simulink model "simple_cosimulation"  (R2021b)
settings: Solver=ode45  StartTime=0.0  StopTime=15  FixedStep=0.01  RelTol=1e-3  EnableMultiTasking=on
libraries: instrumentlib x2, simulink x1
settings Model: PacingRate=11  Creator=tasora  LastModifiedBy=Trevor
settings SolverCC: AlgebraicLoopSolver=TrustRegion
settings DataIOCC: LimitDataPoints=on  SaveFormat=Array  SignalLoggingSaveFormat=ModelDataLogs  ReturnWorkspaceOutputs=off
settings OptimizationCC: ExpressionDepthLimit=2147483647  LifeSpan=inf
settings DebuggingCC: UnderspecifiedInitializationDetection=Classic  MergeDetectMultiDrivingBlocksExec=none  SolverPrmCheckMsg=warning  FcnCallInpInsideContextMsg=warning  StateNameClashWarn=warning  SFUnexpectedBacktrackingDiag=warning  SFNoUnconditionalDefaultTransitionDiag=warning  SFExecutionAtInitializationDiag=none  SFMachineParentedDataDiag=warning  ArithmeticOperatorsInVariantConditions=warning
settings HardwareCC: ProdBitPerPointer=32  ProdBitPerSizeT=32  ProdBitPerPtrDiffT=32  ProdLargestAtomicFloat=None  ProdIntDivRoundTo=Undefined  ProdEndianess=Unspecified  ProdWordSize=32  ProdHWDeviceType=32-bit Generic
settings ModelReferenceCC: PropagateSignalLabelsOutOfModel=off
settings SFSimCC: SimUseLocalCustomCode=off  CustomCodeUndefinedFunction=UseInterfaceOnly
settings RTWCC: RTWUseLocalCustomCode=off
settings CodeAppCC: StateflowObjectComments=on
settings GRTTargetCC: TargetLangStandard=C89/C90 (ANSI)  CombineOutputUpdateFcns=off  GRTInterface=on
settings ConfigComp: CovMetricSettings=dw  CovSaveCumulativeToWorkspaceVar=on  CovSaveSingleToWorkspaceVar=on  CovExternalEMLEnable=off

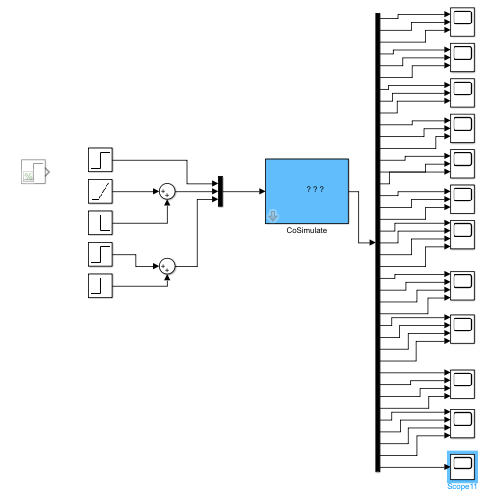
[thumbnail: Simulink's stored preview of the top-level diagram]
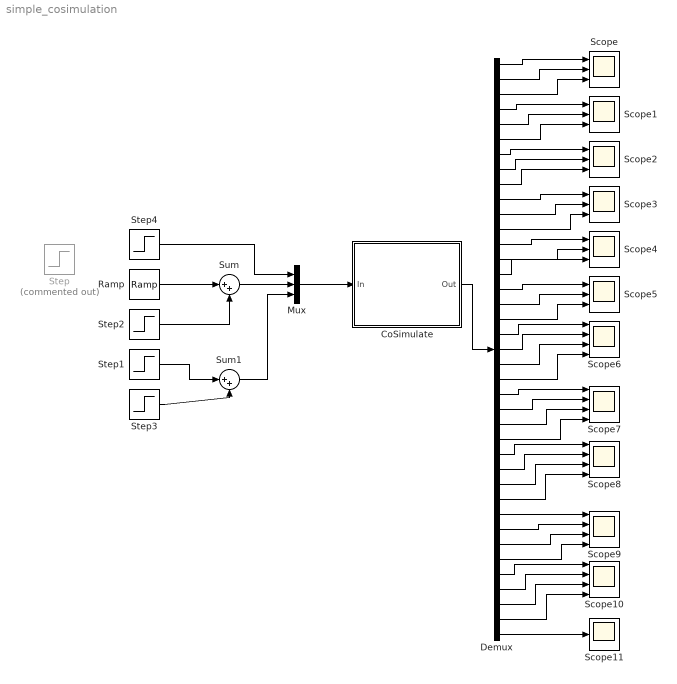
== system simple_cosimulation ==
  CoSimulate : Subsystem  Description=|  mask{com_step=1e-2, tcp_data_size=39, host_name=localhost, tcp_port=50009, tcp_timeout=5}
      | This block can be used to exchange data with Chrono::Engine.                                                                                      
      | A Chrono::Engine program with a running ChCosimulation inferface must be started, it will work as a server; then the Simulink program must be run.
      | Note! check that the dimensions of the exchanged vectors do match!
      mask prompts: com_step "Communication step size"; tcp_data_size "N. of scalars received from C::E (as block output)"; host_name "TCP host name (ex. 'localhost', or 'www.myhost.com')"; tcp_port "TCP port (ex. 50007)"; tcp_timeout "TCP timeout (seconds)"
      mask init:
      | block_receive = [gcb, '/TCP Receive'];
      | set_param(block_receive, 'SampleTime', num2str(com_step));
      | set_param(block_receive, 'Host', host_name);
      | set_param(block_receive, 'Port', num2str(tcp_port));
      | set_param(block_receive, 'DataSize', num2str(tcp_data_size+1));
      | set_param(block_receive, 'Timeout', num2str(tcp_timeout));
      | block_send = [gcb, '/TCP Send'];
      | set_param(block_send, 'Host', host_name);
      | set_param(block_send, 'Port', num2str(tcp_port));
      mask Display:
      | image(imread('block_logo.png'))
      | disp('C::E                   ')
  Demux : Demux  Outputs=39
  Mux : Mux  Inputs=3
  Ramp : simulink/Sources/Ramp  slope=0.1  start=4  InitialOutput=0
  Scope{,1..5} (6 alike) : Scope  NumInputPorts=3
  Scope{6..10} (5 alike) : Scope  NumInputPorts=4
  Scope11 : Scope
  Step : Step  Commented=on  Time=5  SampleTime=0
  Step1 : Step  Time=14  After=0.5  SampleTime=0
  Step2 : Step  Time=12  After=-1  SampleTime=0
  Step3 : Step  Time=0  After=0  SampleTime=0
  Step4 : Step  Time=4  After=0.5  SampleTime=0
  Sum : Sum  Inputs=|++
  Sum1 : Sum  Inputs=|++
  wires:
  Step4/1 -> Mux/1
  Ramp/1 -> Sum/1
  Step1/1 -> Sum1/1
  Mux/1 -> CoSimulate/1(In)
  CoSimulate/1(Out) -> Demux/1
  Demux/1 -> Scope/1
  Demux/2 -> Scope/2
  Demux/3 -> Scope/3
  Demux/4 -> Scope1/1
  Demux/5 -> Scope1/2
  Demux/6 -> Scope1/3
  Demux/7 -> Scope2/1
  Demux/8 -> Scope2/2
  Demux/9 -> Scope2/3
  Demux/10 -> Scope3/1
  Demux/11 -> Scope3/2
  Demux/12 -> Scope3/3
  Demux/14 -> Scope4/2
  Demux/13 -> Scope4/1
  Demux/15 -> Scope4/3
  Demux/17 -> Scope5/2
  Demux/16 -> Scope5/1
  Demux/18 -> Scope5/3
  Step2/1 -> Sum/2
  Sum/1 -> Mux/2
  Step3/1 -> Sum1/2
  Sum1/1 -> Mux/3
  Demux/19 -> Scope6/1
  Demux/20 -> Scope6/2
  Demux/21 -> Scope6/3
  Demux/22 -> Scope6/4
  Demux/23 -> Scope7/1
  Demux/24 -> Scope7/2
  Demux/25 -> Scope7/3
  Demux/26 -> Scope7/4
  Demux/27 -> Scope8/1
  Demux/28 -> Scope8/2
  Demux/29 -> Scope8/3
  Demux/30 -> Scope8/4
  Demux/31 -> Scope9/1
  Demux/32 -> Scope9/2
  Demux/33 -> Scope9/3
  Demux/34 -> Scope9/4
  Demux/35 -> Scope10/1
  Demux/36 -> Scope10/2
  Demux/37 -> Scope10/3
  Demux/38 -> Scope10/4
  Demux/39 -> Scope11/1

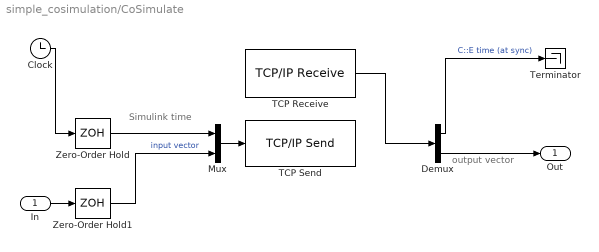
== system simple_cosimulation/CoSimulate ==
  note: output vector
  note: Simulink time
  In : Inport
  Clock : Clock
  Demux : Demux  Outputs=[1 -1]
  Mux : Mux  Inputs=2
  TCP Receive : instrumentlib/TCP//IP Receive  Priority=1  Host=localhost  Port=50009  DataSize=40  DataType=double  ASCIIFormatting=%f  Terminator=LF  CustomTerminator=10  ByteOrder=little-endian  EnableBlockingMode=on  Timeout=5  SampleTime=0.01  SimulateUsing=Interpreted execution
  TCP Send : instrumentlib/TCP//IP Send  Priority=2  Host=localhost  Port=50009  ByteOrder=little-endian  EnableBlockingMode=off  Timeout=10  TransferDelay=on  SimulateUsing=Interpreted execution
  Terminator : Terminator
  Zero-Order Hold : ZeroOrderHold  SampleTime=com_step
  Zero-Order Hold1 : ZeroOrderHold  SampleTime=com_step
  Out : Outport
  wires:
  Zero-Order Hold/1 -> Mux/1
  Zero-Order Hold1/1 -> Mux/2  "input vector"
  Mux/1 -> TCP Send/1
  Clock/1 -> Zero-Order Hold/1
  In/1 -> Zero-Order Hold1/1
  TCP Receive/1 -> Demux/1
  Demux/1 -> Terminator/1  "C::E time (at sync)"
  Demux/2 -> Out/1
